simulink model "main"  (R2021b)
settings: Solver=ode1be  StartTime=0.0  StopTime=20  FixedStep=0.001  RelTol=1e-3
undefined symbols (not defined in the file): X, Y, Z
libraries: sm_lib x5, robotics_pg_exp_pack x4, nesl_utility x1
settings Model: Creator=zyr77  LastModifiedBy=zyr77
settings ExplorerConfigSet: InternalSimMechanicsExplorerSettings="<ExplorerConfiguration><canonicalview>default</canonicalview><AnimationSetting><BasePlaybackSpeed>1.0</BasePlaybackSpeed><PlaybackSpeedFactor>1.0</PlaybackSpeedFactor></AnimationSetting><TilePanel><TileInfo><Tiles Columns=\"1\" Count=\"1\" Rows=\"1\"><Column Weight=\"1\"/><Row Weight=\"1\"/><Tile Height=\"1\" Width=\"1\" X=\"0\" Y=\"0\"/></Tiles></TileInfo><SceneInfo><SceneViewer><BGColor><R>0.60000002384185791</R><G>0.60000002384185791</G><B>0.60000002384185791</B></BGColor><Camera><DoPerspective>off</DoPerspective><Position><X>10.6873296003530456</X><Y>-7.40477011556181708</Y><Z>18.8477519699292095</Z></Position><Center><X>10.1085197213467506</X><Y>0.00225702434517494055</Y><Z>-1.20402255587443818</Z></Center><Up><X>0.00801237773987227564</X><Y>0.938091421695407712</Y><Z>0.346295085648702816</Z></Up><ViewLimDist>1</ViewLimDist><YLim>14.8793175993082993</YLim><XLim>21.5701267167215498</XLim></Camera></SceneViewer></SceneInfo></TilePanel><MechEditorPanel><Cameras/><GfxPanelCameraMap/><VideoCreator><PlaybackSpeedRatio>1.0</PlaybackSpeedRatio><FrameRate>60</FrameRate><VideoFormat>MPEG-4</VideoFormat><FrameSize>[1920 1080]</FrameSize></VideoCreator></MechEditorPanel></ExplorerConfiguration>"

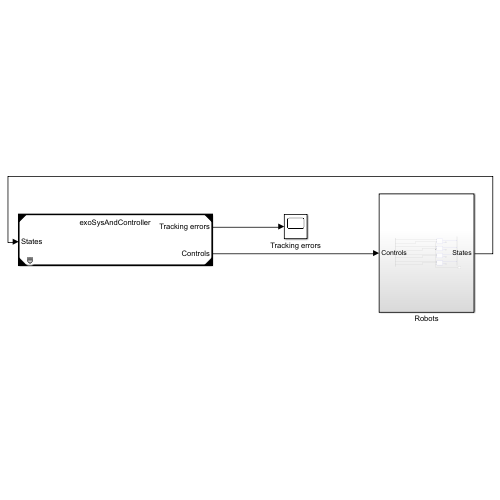
[thumbnail: Simulink's stored preview of the top-level diagram]
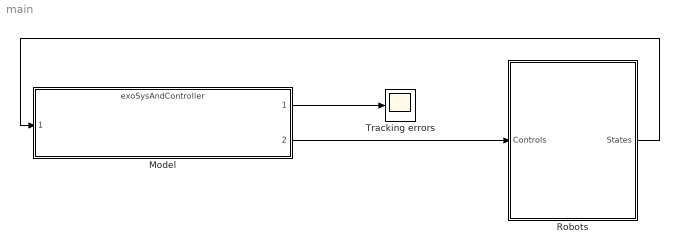
== system main ==
  Model : ModelReference  ModelNameDialog=exoSysAndController.slxp  ModelReferenceVersion=1.423  CopyOfModelProtected=on
  Robots : Subsystem
  Tracking errors : Scope
  wires:
  Model/2 -> Robots/1(Controls)
  Robots/1(States) -> Model/1
  Model/1 -> Tracking errors/1

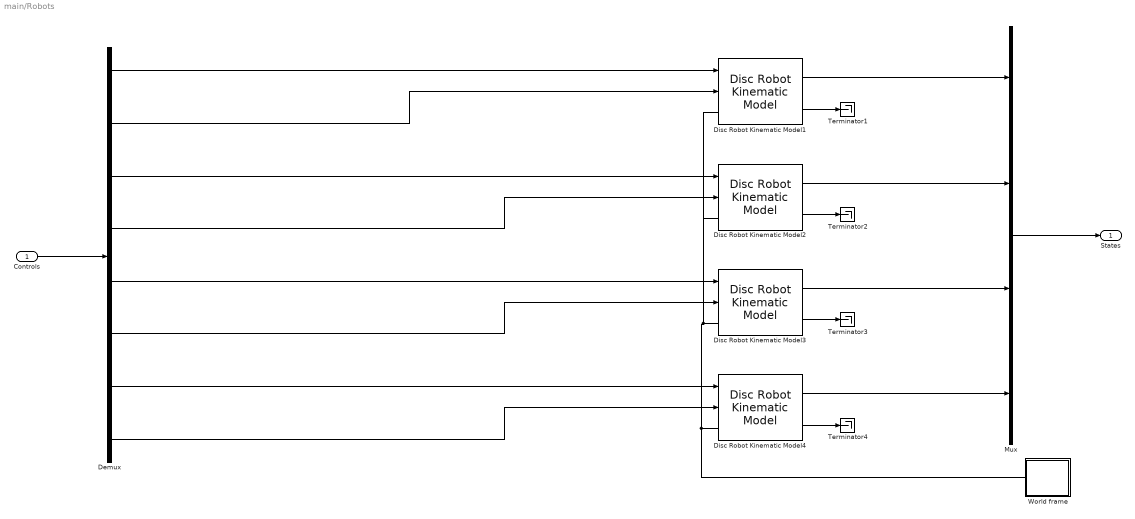
== system main/Robots ==
  Controls : Inport
  Demux : Demux  Outputs=8
  Disc Robot Kinematic Model1 : robotics_pg_exp_pack/Robot Models/MATLAB Disc Robot/Disc Robot Kinematic Model  robotId=1  wheelRadius=0.3  wheelBase=1  wheelThickness=0.025  chassisThickness=0.05  startPose=[0 -1 0]  choice=off  sensorTs=0.001  wheelColor=[0.25 0.25 0.25]  chassisColor=[0.5 0.25 0.25]
      settings: SourceProductName=Robotics Playground Expansion Pack
  Disc Robot Kinematic Model2 : robotics_pg_exp_pack/Robot Models/MATLAB Disc Robot/Disc Robot Kinematic Model  robotId=1  wheelRadius=0.3  wheelBase=1  wheelThickness=0.025  chassisThickness=0.05  startPose=[-1 1 0]  choice=off  sensorTs=0.001  wheelColor=[0.25 0.25 0.25]  chassisColor=[0.4 0.6 0.8]
      settings: SourceProductName=Robotics Playground Expansion Pack
  Disc Robot Kinematic Model3 : robotics_pg_exp_pack/Robot Models/MATLAB Disc Robot/Disc Robot Kinematic Model  robotId=1  wheelRadius=0.3  wheelBase=1  wheelThickness=0.025  chassisThickness=0.05  startPose=[-3 1 0]  choice=off  sensorTs=0.001  wheelColor=[0.25 0.25 0.25]  chassisColor=[0.2 0.9 0.8]
      settings: SourceProductName=Robotics Playground Expansion Pack
  Disc Robot Kinematic Model4 : robotics_pg_exp_pack/Robot Models/MATLAB Disc Robot/Disc Robot Kinematic Model  robotId=1  wheelRadius=0.3  wheelBase=1  wheelThickness=0.025  chassisThickness=0.05  startPose=[2 -1 0]  choice=off  sensorTs=0.001  wheelColor=[0.25 0.25 0.25]  chassisColor=[0.9 0.1 0.2]
      settings: SourceProductName=Robotics Playground Expansion Pack
  Mux : Mux
  Terminator{1..4} (4 alike) : Terminator
  World frame : Subsystem
  States : Outport
  wires:
  Disc Robot Kinematic Model2/2 -> Terminator2/1
  Disc Robot Kinematic Model4/2 -> Terminator4/1
  Disc Robot Kinematic Model1/2 -> Terminator1/1
  Disc Robot Kinematic Model3/2 -> Terminator3/1
  Demux/5 -> Disc Robot Kinematic Model3/1
  Demux/7 -> Disc Robot Kinematic Model4/1
  Demux/8 -> Disc Robot Kinematic Model4/2
  Disc Robot Kinematic Model4/1 -> Mux/4
  Disc Robot Kinematic Model3/1 -> Mux/3
  Demux/6 -> Disc Robot Kinematic Model3/2
  Demux/2 -> Disc Robot Kinematic Model1/2
  Demux/1 -> Disc Robot Kinematic Model1/1
  Disc Robot Kinematic Model1/1 -> Mux/1
  Demux/4 -> Disc Robot Kinematic Model2/2
  Demux/3 -> Disc Robot Kinematic Model2/1
  Disc Robot Kinematic Model2/1 -> Mux/2
  Controls/1 -> Demux/1
  Mux/1 -> States/1
  connections:
  Disc Robot Kinematic Model3/LConn1 -- Disc Robot Kinematic Model1/LConn1 -- Disc Robot Kinematic Model2/LConn1 -- Disc Robot Kinematic Model4/LConn1 -- World frame/LConn1

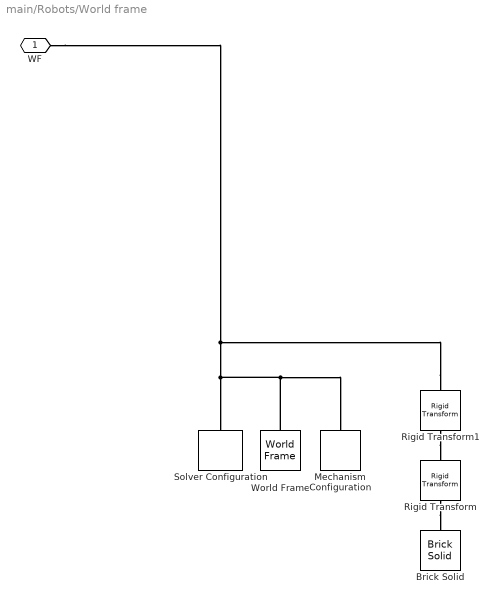
== system main/Robots/World frame ==
  Brick Solid : sm_lib/Body Elements/Brick Solid  GraphicAmbientColor=[0.15 0.15 0.15 1.0]  BasedOnType=Density  BrickDimensions=[40 10 1]  BrickDimensionUnits=m  CenterOfMass=[0 0 0]  CenterOfMassUnits=m  GraphicDiffuseColor=[0.8 0.8 0.8]  Density=1000  DensityUnits=kg/m^3  DoExposeReferenceFrame=on  GraphicEmissiveColor=[0.0 0.0 0.0 1.0]  ExportEntireGeometry=off  SerializedFrames=<Frames/>  MarkerShape=Sphere  MarkerSize=10  GraphicType=FromGeometry  InertiaType=CalculateFromGeometry  Mass=1  MassUnits=kg  MomentsOfInertia=[1 1 1]  MomentsOfInertiaUnits=kg*m^2  GraphicOpacity=1.0  ProductsOfInertia=[0 0 0]  ProductsOfInertiaUnits=kg*m^2  GraphicShininess=75  GraphicSpecularColor=[0.5 0.5 0.5 1.0]  GraphicVisPropType=SimpleVisualProperties
  Mechanism Configuration : sm_lib/Utilities/Mechanism Configuration  UniformGravity=Constant  GravityVector=[0 0 -9.80665]  GravityUnits=m/s^2  LinearizationDelta=0.001  JointModeTransitionNonlinearIterations=2
  Rigid Transform : sm_lib/Frames and Transforms/Rigid Transform  TranslationMethod=StandardAxis  TranslationStandardOffset=0.5  TranslationLengthUnit=m  TranslationStandardAxis=+Z  TranslationCartesianOffset=[0 0 0]  TranslationROffset=0  TranslationROffsetUnits=m  TranslationZOffset=0  TranslationZOffsetUnits=m  TranslationThetaOffset=0  TranslationThetaOffsetUnits=deg  RotationMethod=None  RotationAngleUnits=deg  RotationStandardAxis=+Z  RotationAngle=0.0  RotationArbitraryAxis=[0 0 1]  FollAlignAxisA=+X  BaseAlignAxisA=+Y  FollAlignAxisB=+Y  BaseAlignAxisB=+Z  RotationSequenceAxes=FollowerAxes  RotationSequence=XYX  RotationSequenceAngles=[0 0 0]  RotationSequenceAnglesUnits=deg  RotationMatrix=[1 0 0; 0 1 0; 0 0 1]
  Rigid Transform1 : sm_lib/Frames and Transforms/Rigid Transform  TranslationMethod=StandardAxis  TranslationStandardOffset=10  TranslationLengthUnit=m  TranslationStandardAxis=-X  TranslationCartesianOffset=[0 0 0]  TranslationROffset=0  TranslationROffsetUnits=m  TranslationZOffset=0  TranslationZOffsetUnits=m  TranslationThetaOffset=0  TranslationThetaOffsetUnits=deg  RotationMethod=None  RotationAngleUnits=deg  RotationStandardAxis=+Z  RotationAngle=0.0  RotationArbitraryAxis=[0 0 1]  FollAlignAxisA=+X  BaseAlignAxisA=+Y  FollAlignAxisB=+Y  BaseAlignAxisB=+Z  RotationSequenceAxes=FollowerAxes  RotationSequence=XYX  RotationSequenceAngles=[0 0 0]  RotationSequenceAnglesUnits=deg  RotationMatrix=[1 0 0; 0 1 0; 0 0 1]
  Solver Configuration : nesl_utility/Solver Configuration  PhysicalDomain=network_engine_domain  SubClassName=solver  LeftPortType=input  RightPortType=generic  Tones=[]  Harmonics=[]  SimulateNoise=off  Profile=off  UseLocalSampling=off  EnableSwitchedLinearOptims=on  FrequencyDomain=off  UseCCode=off  RelTol=0.001  AbsTol=1e-06  MinStep=1e-09  ToWorkspace=off  RevertToSquareIcSolve=off  NumHomotopyIterations=100  PhasorMode=off  PhasorModeNumHarmonics=1  DoDC=off  ResidualTolerance=1e-09  UseLocalSolver=off  LocalSolverChoice=NE_BACKWARD_EULER_ADVANCER  LocalSolverSampleTime=0.001  DoFixedCost=off  MaxNonlinIter=3  MaxModeIter=2  ComputeImpulses=off  ImpulseIterations=2  LinearAlgebra=auto  EquationFormulation=NE_TIME_EF  DelaysMemoryBudget=1024  AutomaticFiltering=on  FilteringTimeConstant=0.001  PartitionStorageMethod=AS_NEEDED  PartitionMemoryBudget=1024  PartitionMethod=ROBUST
      settings: SourceProductBaseCode=PW,SS
  World Frame : sm_lib/Frames and Transforms/World Frame
  WF : PMIOPort  Side=Left
  connections:
  Rigid Transform/LConn1 -- Brick Solid/RConn1
  Rigid Transform1/RConn1 -- WF/RConn1 -- World Frame/RConn1 -- Mechanism Configuration/RConn1 -- Solver Configuration/RConn1
  Rigid Transform1/LConn1 -- Rigid Transform/RConn1
